simulink model "Modelo8_Harness1"  (R2020b)
settings: Solver=FixedStepAuto  StartTime=0.0  StopTime=inf  FixedStep=1e-2  MaxStep=1e-4  RelTol=1e-3
settings Model: Creator=GoniR  LastModifiedBy=GoniR
settings SolverCC: ConcurrentTasks=on  ZeroCrossAlgorithm=Adaptive  AutoInsertRateTranBlk=on
settings DebuggingCC: MaskedZcDiagnostic=none  IgnoredZcDiagnostic=none
settings HardwareCC: ProdHWDeviceType=AMD->x86-64 (Windows64)
settings SFSimCC: SimTargetLang=C++
settings ConfigComp: PLC_TargetIDE=codesys23

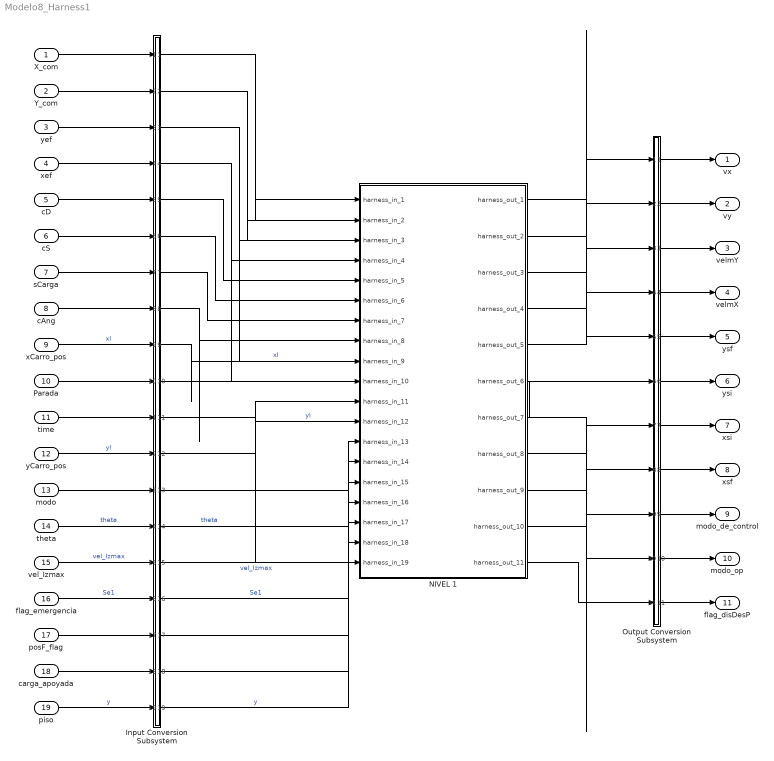
== system Modelo8_Harness1 ==
  X_com : Inport  OutDataTypeStr=double  PortDimensions=[1]  SampleTime=0.01
  Y_com : Inport  Port=2  OutDataTypeStr=double  PortDimensions=[1]  SampleTime=0.01
  yef : Inport  Port=3  OutDataTypeStr=double  PortDimensions=[1]  SampleTime=[-1, 0]
  xef : Inport  Port=4  OutDataTypeStr=double  PortDimensions=[1]  SampleTime=[-1, 0]
  cD : Inport  Port=5  OutDataTypeStr=double  PortDimensions=[1]  SampleTime=0.01
  cS : Inport  Port=6  OutDataTypeStr=double  PortDimensions=[1]  SampleTime=0.01
  sCarga : Inport  Port=7  OutDataTypeStr=double  PortDimensions=[1]  SampleTime=[-1, 0]
  cAng : Inport  Port=8  OutDataTypeStr=double  PortDimensions=[1]  SampleTime=[-1, 0]
  xCarro_pos : Inport  Port=9  OutDataTypeStr=double  PortDimensions=[1]  SampleTime=0
  Parada : Inport  Port=10  OutDataTypeStr=double  PortDimensions=[1]  SampleTime=0.01
  time : Inport  Port=11  OutDataTypeStr=double  PortDimensions=[1]  SampleTime=0
  yCarro_pos : Inport  Port=12  OutDataTypeStr=double  PortDimensions=[1]  SampleTime=0
  modo : Inport  Port=13  OutDataTypeStr=double  PortDimensions=[1]  SampleTime=0.01
  theta : Inport  Port=14  OutDataTypeStr=double  PortDimensions=[1]  SampleTime=0
  vel_Izmax : Inport  Port=15  OutDataTypeStr=double  PortDimensions=[1]  SampleTime=0.01
  flag_emergencia : Inport  Port=16  OutDataTypeStr=double  PortDimensions=[1]  SampleTime=0.01
  posF_flag : Inport  Port=17  OutDataTypeStr=double  PortDimensions=[1]  SampleTime=[-1, 0]
  carga_apoyada : Inport  Port=18  OutDataTypeStr=double  PortDimensions=[1]  SampleTime=0
  piso : Inport  Port=19  OutDataTypeStr=double  PortDimensions=[1]  SampleTime=0
  Input Conversion Subsystem : Subsystem  Tag=__SLT_ICS__  Description=|
      | Signal spec.
      | and routing
      settings: AttributesFormatString=%<Description>
  NIVEL 1 : Subsystem  Tag=__SL_testing_harness_stub_
  Output Conversion Subsystem : Subsystem  Tag=__SLT_OCS__  Description=|
      | Signal spec.
      | and routing
      settings: AttributesFormatString=%<Description>
  vx : Outport
  vy : Outport  Port=2
  velmY : Outport  Port=3
  velmX : Outport  Port=4
  ysf : Outport  Port=5
  ysi : Outport  Port=6
  xsi : Outport  Port=7
  xsf : Outport  Port=8
  modo_de_control : Outport  Port=9
  modo_op : Outport  Port=10
  flag_disDesP : Outport  Port=11
  wires:
  X_com/1 -> Input Conversion Subsystem/1(Inport_1)
  Y_com/1 -> Input Conversion Subsystem/2(Inport_2)
  yef/1 -> Input Conversion Subsystem/3(Inport_3)
  xef/1 -> Input Conversion Subsystem/4(Inport_4)
  cD/1 -> Input Conversion Subsystem/5(Inport_5)
  cS/1 -> Input Conversion Subsystem/6(Inport_6)
  sCarga/1 -> Input Conversion Subsystem/7(Inport_7)
  cAng/1 -> Input Conversion Subsystem/8(Inport_8)
  xCarro_pos/1 -> Input Conversion Subsystem/9(Inport_9)  "xl"
  Parada/1 -> Input Conversion Subsystem/10(Inport_10)
  time/1 -> Input Conversion Subsystem/11(Inport_11)
  yCarro_pos/1 -> Input Conversion Subsystem/12(Inport_12)  "yl"
  modo/1 -> Input Conversion Subsystem/13(Inport_13)
  theta/1 -> Input Conversion Subsystem/14(Inport_14)  "theta"
  vel_Izmax/1 -> Input Conversion Subsystem/15(Inport_15)  "vel_Izmax"
  flag_emergencia/1 -> Input Conversion Subsystem/16(Inport_16)  "Se1"
  posF_flag/1 -> Input Conversion Subsystem/17(Inport_17)
  carga_apoyada/1 -> Input Conversion Subsystem/18(Inport_18)
  piso/1 -> Input Conversion Subsystem/19(Inport_19)  "y"
  Output Conversion Subsystem/1(Outport_1) -> vx/1
  Output Conversion Subsystem/2(Outport_2) -> vy/1
  Output Conversion Subsystem/3(Outport_3) -> velmY/1
  Output Conversion Subsystem/4(Outport_4) -> velmX/1
  Output Conversion Subsystem/5(Outport_5) -> ysf/1
  Output Conversion Subsystem/6(Outport_6) -> ysi/1
  Output Conversion Subsystem/7(Outport_7) -> xsi/1
  Output Conversion Subsystem/8(Outport_8) -> xsf/1
  Output Conversion Subsystem/9(Outport_9) -> modo_de_control/1
  Output Conversion Subsystem/10(Outport_10) -> modo_op/1
  Output Conversion Subsystem/11(Outport_11) -> flag_disDesP/1
  Input Conversion Subsystem/1(Outport_1) -> NIVEL 1/1(harness_in_1)
  Input Conversion Subsystem/2(Outport_2) -> NIVEL 1/2(harness_in_2)
  Input Conversion Subsystem/3(Outport_3) -> NIVEL 1/3(harness_in_3)
  Input Conversion Subsystem/4(Outport_4) -> NIVEL 1/4(harness_in_4)
  Input Conversion Subsystem/5(Outport_5) -> NIVEL 1/5(harness_in_5)
  Input Conversion Subsystem/6(Outport_6) -> NIVEL 1/6(harness_in_6)
  Input Conversion Subsystem/7(Outport_7) -> NIVEL 1/7(harness_in_7)
  Input Conversion Subsystem/8(Outport_8) -> NIVEL 1/8(harness_in_8)
  Input Conversion Subsystem/9(Outport_9) -> NIVEL 1/9(harness_in_9)  "xl"
  Input Conversion Subsystem/10(Outport_10) -> NIVEL 1/10(harness_in_10)
  Input Conversion Subsystem/11(Outport_11) -> NIVEL 1/11(harness_in_11)
  Input Conversion Subsystem/12(Outport_12) -> NIVEL 1/12(harness_in_12)  "yl"
  Input Conversion Subsystem/13(Outport_13) -> NIVEL 1/13(harness_in_13)
  Input Conversion Subsystem/14(Outport_14) -> NIVEL 1/14(harness_in_14)  "theta"
  Input Conversion Subsystem/15(Outport_15) -> NIVEL 1/15(harness_in_15)  "vel_Izmax"
  Input Conversion Subsystem/16(Outport_16) -> NIVEL 1/16(harness_in_16)  "Se1"
  Input Conversion Subsystem/17(Outport_17) -> NIVEL 1/17(harness_in_17)
  Input Conversion Subsystem/18(Outport_18) -> NIVEL 1/18(harness_in_18)
  Input Conversion Subsystem/19(Outport_19) -> NIVEL 1/19(harness_in_19)  "y"
  NIVEL 1/1(harness_out_1) -> Output Conversion Subsystem/1(Inport_1)
  NIVEL 1/2(harness_out_2) -> Output Conversion Subsystem/2(Inport_2)
  NIVEL 1/3(harness_out_3) -> Output Conversion Subsystem/3(Inport_3)
  NIVEL 1/4(harness_out_4) -> Output Conversion Subsystem/4(Inport_4)
  NIVEL 1/5(harness_out_5) -> Output Conversion Subsystem/5(Inport_5)
  NIVEL 1/6(harness_out_6) -> Output Conversion Subsystem/6(Inport_6)
  NIVEL 1/7(harness_out_7) -> Output Conversion Subsystem/7(Inport_7)
  NIVEL 1/8(harness_out_8) -> Output Conversion Subsystem/8(Inport_8)
  NIVEL 1/9(harness_out_9) -> Output Conversion Subsystem/9(Inport_9)
  NIVEL 1/10(harness_out_10) -> Output Conversion Subsystem/10(Inport_10)
  NIVEL 1/11(harness_out_11) -> Output Conversion Subsystem/11(Inport_11)

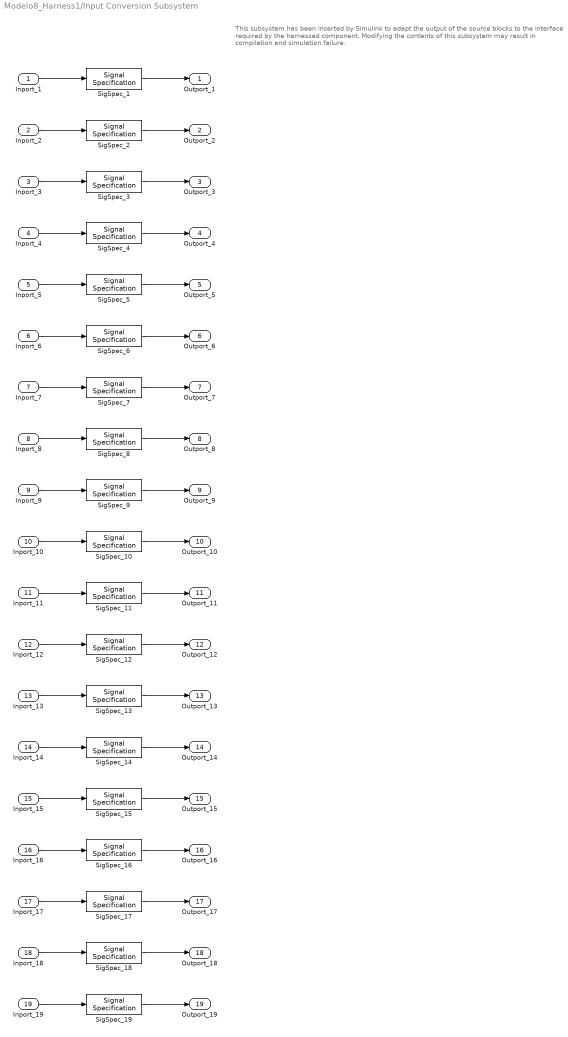
== system Modelo8_Harness1/Input Conversion Subsystem ==
  note: This subsystem has been inserted by Simulink to adapt the output of the source blocks to the interface required by the harnessed component.
      |  Modifying the contents of this subsystem may result in compilation and simulation failure.
  Inport_1 : Inport
  Inport_2 : Inport  Port=2
  Inport_3 : Inport  Port=3
  Inport_4 : Inport  Port=4
  Inport_5 : Inport  Port=5
  Inport_6 : Inport  Port=6
  Inport_7 : Inport  Port=7
  Inport_8 : Inport  Port=8
  Inport_9 : Inport  Port=9
  Inport_10 : Inport  Port=10
  Inport_11 : Inport  Port=11
  Inport_12 : Inport  Port=12
  Inport_13 : Inport  Port=13
  Inport_14 : Inport  Port=14
  Inport_15 : Inport  Port=15
  Inport_16 : Inport  Port=16
  Inport_17 : Inport  Port=17
  Inport_18 : Inport  Port=18
  Inport_19 : Inport  Port=19
  SigSpec_{1..2,5..6,10,13,15..16} (8 alike) : SignalSpecification  OutDataTypeStr=double  Dimensions=[1]  SampleTime=0.01
  SigSpec_{9,11..12,14,18..19} (6 alike) : SignalSpecification  OutDataTypeStr=double  Dimensions=[1]  SampleTime=[0, 0]
  SigSpec_{3..4,7..8,17} (5 alike) : SignalSpecification  OutDataTypeStr=double  Dimensions=[1]  SampleTime=[-1, 0]
  Outport_1 : Outport
  Outport_2 : Outport  Port=2
  Outport_3 : Outport  Port=3
  Outport_4 : Outport  Port=4
  Outport_5 : Outport  Port=5
  Outport_6 : Outport  Port=6
  Outport_7 : Outport  Port=7
  Outport_8 : Outport  Port=8
  Outport_9 : Outport  Port=9
  Outport_10 : Outport  Port=10
  Outport_11 : Outport  Port=11
  Outport_12 : Outport  Port=12
  Outport_13 : Outport  Port=13
  Outport_14 : Outport  Port=14
  Outport_15 : Outport  Port=15
  Outport_16 : Outport  Port=16
  Outport_17 : Outport  Port=17
  Outport_18 : Outport  Port=18
  Outport_19 : Outport  Port=19
  wires:
  SigSpec_1/1 -> Outport_1/1
  Inport_1/1 -> SigSpec_1/1
  SigSpec_2/1 -> Outport_2/1
  Inport_2/1 -> SigSpec_2/1
  SigSpec_3/1 -> Outport_3/1
  Inport_3/1 -> SigSpec_3/1
  SigSpec_4/1 -> Outport_4/1
  Inport_4/1 -> SigSpec_4/1
  SigSpec_5/1 -> Outport_5/1
  Inport_5/1 -> SigSpec_5/1
  SigSpec_6/1 -> Outport_6/1
  Inport_6/1 -> SigSpec_6/1
  SigSpec_7/1 -> Outport_7/1
  Inport_7/1 -> SigSpec_7/1
  SigSpec_8/1 -> Outport_8/1
  Inport_8/1 -> SigSpec_8/1
  SigSpec_9/1 -> Outport_9/1
  Inport_9/1 -> SigSpec_9/1
  SigSpec_10/1 -> Outport_10/1
  Inport_10/1 -> SigSpec_10/1
  SigSpec_11/1 -> Outport_11/1
  Inport_11/1 -> SigSpec_11/1
  SigSpec_12/1 -> Outport_12/1
  Inport_12/1 -> SigSpec_12/1
  SigSpec_13/1 -> Outport_13/1
  Inport_13/1 -> SigSpec_13/1
  SigSpec_14/1 -> Outport_14/1
  Inport_14/1 -> SigSpec_14/1
  SigSpec_15/1 -> Outport_15/1
  Inport_15/1 -> SigSpec_15/1
  SigSpec_16/1 -> Outport_16/1
  Inport_16/1 -> SigSpec_16/1
  SigSpec_17/1 -> Outport_17/1
  Inport_17/1 -> SigSpec_17/1
  SigSpec_18/1 -> Outport_18/1
  Inport_18/1 -> SigSpec_18/1
  SigSpec_19/1 -> Outport_19/1
  Inport_19/1 -> SigSpec_19/1

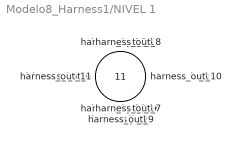
== system Modelo8_Harness1/NIVEL 1 ==
  harness_in_1 : Inport
  harness_in_2 : Inport  Port=2
  harness_in_3 : Inport  Port=3
  harness_in_4 : Inport  Port=4
  harness_in_5 : Inport  Port=5
  harness_in_6 : Inport  Port=6
  harness_in_7 : Inport  Port=7
  harness_in_8 : Inport  Port=8
  harness_in_9 : Inport  Port=9
  harness_in_10 : Inport  Port=10
  harness_in_11 : Inport  Port=11
  harness_in_12 : Inport  Port=12
  harness_in_13 : Inport  Port=13
  harness_in_14 : Inport  Port=14
  harness_in_15 : Inport  Port=15
  harness_in_16 : Inport  Port=16
  harness_in_17 : Inport  Port=17
  harness_in_18 : Inport  Port=18
  harness_in_19 : Inport  Port=19
  harness_out_1 : Outport
  harness_out_2 : Outport  Port=2
  harness_out_3 : Outport  Port=3
  harness_out_4 : Outport  Port=4
  harness_out_5 : Outport  Port=5
  harness_out_6 : Outport  Port=6
  harness_out_7 : Outport  Port=7
  harness_out_8 : Outport  Port=8
  harness_out_9 : Outport  Port=9
  harness_out_10 : Outport  Port=10
  harness_out_11 : Outport  Port=11

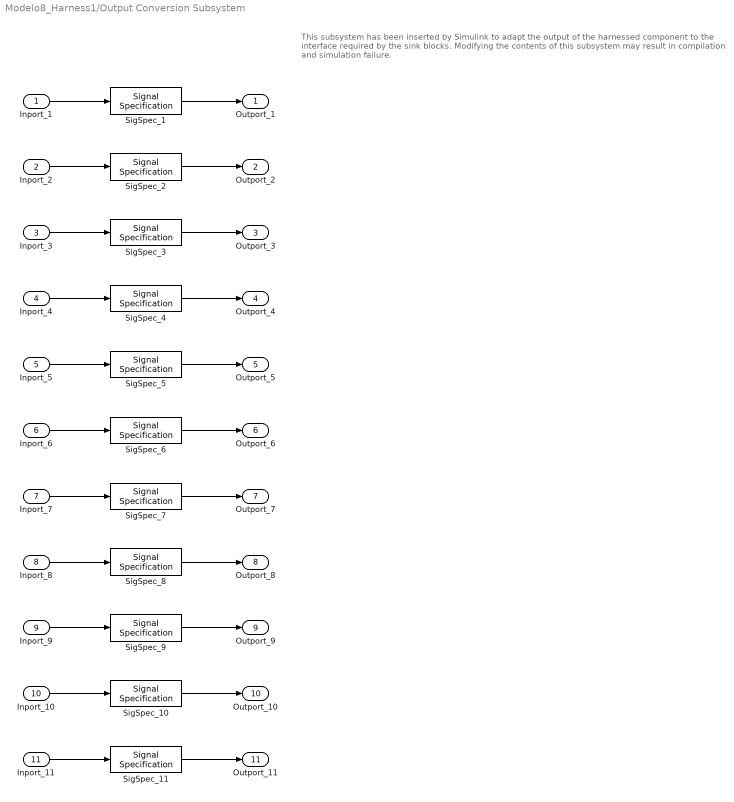
== system Modelo8_Harness1/Output Conversion Subsystem ==
  note: This subsystem has been inserted by Simulink to adapt the output of the harnessed component to the interface required by the sink blocks.
      |  Modifying the contents of this subsystem may result in compilation and simulation failure.
  Inport_1 : Inport
  Inport_2 : Inport  Port=2
  Inport_3 : Inport  Port=3
  Inport_4 : Inport  Port=4
  Inport_5 : Inport  Port=5
  Inport_6 : Inport  Port=6
  Inport_7 : Inport  Port=7
  Inport_8 : Inport  Port=8
  Inport_9 : Inport  Port=9
  Inport_10 : Inport  Port=10
  Inport_11 : Inport  Port=11
  SigSpec_{1..8,10..11} (10 alike) : SignalSpecification  OutDataTypeStr=double  Dimensions=[1]  SampleTime=0.01
  SigSpec_9 : SignalSpecification  OutDataTypeStr=double  Dimensions=[1, 1]  SampleTime=0.01
  Outport_1 : Outport
  Outport_2 : Outport  Port=2
  Outport_3 : Outport  Port=3
  Outport_4 : Outport  Port=4
  Outport_5 : Outport  Port=5
  Outport_6 : Outport  Port=6
  Outport_7 : Outport  Port=7
  Outport_8 : Outport  Port=8
  Outport_9 : Outport  Port=9
  Outport_10 : Outport  Port=10
  Outport_11 : Outport  Port=11
  wires:
  Inport_1/1 -> SigSpec_1/1
  SigSpec_1/1 -> Outport_1/1
  Inport_2/1 -> SigSpec_2/1
  SigSpec_2/1 -> Outport_2/1
  Inport_3/1 -> SigSpec_3/1
  SigSpec_3/1 -> Outport_3/1
  Inport_4/1 -> SigSpec_4/1
  SigSpec_4/1 -> Outport_4/1
  Inport_5/1 -> SigSpec_5/1
  SigSpec_5/1 -> Outport_5/1
  Inport_6/1 -> SigSpec_6/1
  SigSpec_6/1 -> Outport_6/1
  Inport_7/1 -> SigSpec_7/1
  SigSpec_7/1 -> Outport_7/1
  Inport_8/1 -> SigSpec_8/1
  SigSpec_8/1 -> Outport_8/1
  Inport_9/1 -> SigSpec_9/1
  SigSpec_9/1 -> Outport_9/1
  Inport_10/1 -> SigSpec_10/1
  SigSpec_10/1 -> Outport_10/1
  Inport_11/1 -> SigSpec_11/1
  SigSpec_11/1 -> Outport_11/1
